simulink subsystem "monitor_simulink"  (R2022b)
settings: Solver=VariableStepAuto  StartTime=0.0  StopTime=10.0  RelTol=1e-3
settings Model: Creator=User  LastModifiedBy=User

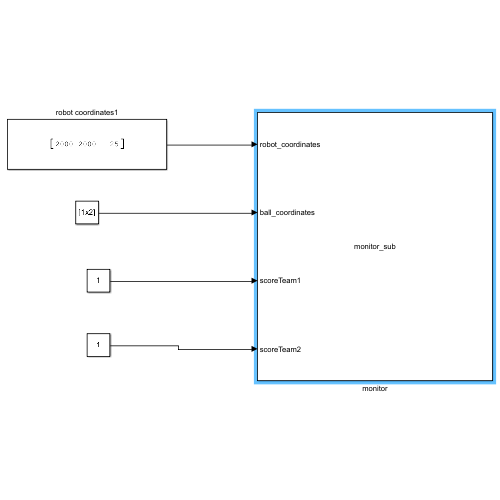
[thumbnail: Simulink's stored preview of the top-level diagram]
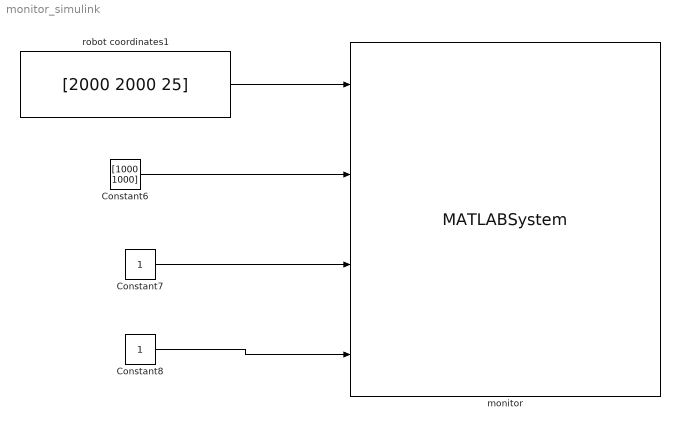
== system monitor_simulink ==
  Constant6 : Constant  Value=[1000 1000]
  Constant7 : Constant
  Constant8 : Constant
  monitor : MATLABSystem  System=monitor_sub  pitch_length=[]  pitch_width=[]  centre_circle_diameter=[]  border_strip_width=[]  goal_area_length=[]  goal_area_width=[]  penalty_area_length=[]  penalty_area_width=[]  goal_width=[]  goal_depth=[]  SimulateUsing=Code generation
      mask Type: monitor_sub
      mask Display:
      | disp('monitor_sub');
      | port_label('input',1,'robot_coordinates');
      | port_label('input',2,'ball_coordinates');
      | port_label('input',3,'scoreTeam1');
      | port_label('input',4,'scoreTeam2');
  robot coordinates1 : Constant  Value=[2000 2000 25]  VectorParams1D=off
  wires:
  Constant6/1 -> monitor/2
  robot coordinates1/1 -> monitor/1
  Constant7/1 -> monitor/3
  Constant8/1 -> monitor/4
